simulink model "gantrycrane_animation2"  (Simulink 8.0)
settings: Solver=ode45  StartTime=0.0  StopTime=30  RelTol=1e-3
values from neighbouring files (symbols this model uses):
  kdth = -2*zetath*wnth*P.mc*P.L    [param.m]
  kdx = -0.0685    [param.m]
  kpth = (P.mc+P.m)*P.g - wnth^2*P.mc*P.L    [param.m]
  kpx = -0.0385    [param.m]
undefined symbols (not defined in the file or in its folder): drawGantryCrane
libraries: simulink x1
settings Model: Creator=nedward  LastModifiedBy=tmclain
settings DataIOCC: SignalLoggingSaveFormat=ModelDataLogs
settings DebuggingCC: FcnCallInpInsideContextMsg=UseLocalSettings
settings GRTTargetCC: CombineOutputUpdateFcns=off  GRTInterface=on

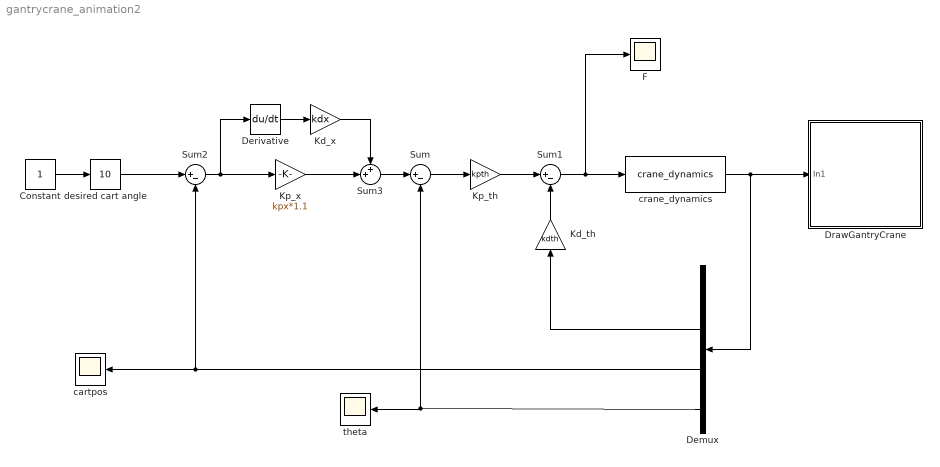
== system gantrycrane_animation2 ==
  Constant : Constant
  Demux : Demux
  Derivative : Derivative
  DrawGantryCrane : Subsystem
      mask init:
      | bar = 20;
      | crane = [5 3];
      | L1 = 10;
      | R1 = 1;
      mask Display: image(imread('tv.jpg'))
  F : Scope
      settings: TimeRange=30  YMin=-2000  YMax=14000  SaveName=ScopeData3
  Kd_th : Gain  Gain=kdth
  Kd_x : Gain  Gain=kdx
  Kp_th : Gain  Gain=kpth
  Kp_x : Gain  Gain=kpx*1.1
  Sum : Sum  Inputs=|+-
  Sum1 : Sum  Inputs=|+-
  Sum2 : Sum  Inputs=|+-
  Sum3 : Sum  Inputs=++|
  cartpos : Scope
      settings: TimeRange=30  YMin=0  YMax=12
  crane_dynamics : S-Function  FunctionName=crane_dynamics  Parameters=P  EnableBusSupport=off
  desired cart angle : simulink/Math Operations/Slider Gain  low=-10  gain=10  high=10
  theta : Scope
      settings: TimeRange=30  YMin=-0.2  YMax=0.15
  wires:
  crane_dynamics/1 -> DrawGantryCrane/1(In1), Demux/1
  Constant/1 -> desired cart angle/1
  Demux/2 -> Kd_th/1
  desired cart angle/1 -> Sum2/1
  Kd_th/1 -> Sum1/2
  Demux/4 -> theta/1, Sum/2
  Sum1/1 -> crane_dynamics/1, F/1
  Demux/3 -> cartpos/1, Sum2/2
  Kp_th/1 -> Sum1/1
  Sum/1 -> Kp_th/1
  Sum3/1 -> Sum/1
  Sum2/1 -> Kp_x/1, Derivative/1
  Kp_x/1 -> Sum3/2
  Derivative/1 -> Kd_x/1
  Kd_x/1 -> Sum3/1

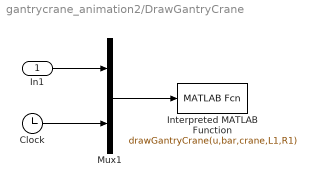
== system gantrycrane_animation2/DrawGantryCrane ==
  In1 : Inport
  Clock : Clock
  Interpreted MATLAB Function : MATLABFcn  MATLABFcn=drawGantryCrane(u,bar,crane,L1,R1)  OutputDimensions=0  SampleTime=0.1
  Mux1 : Mux  Inputs=2
  wires:
  Clock/1 -> Mux1/2
  Mux1/1 -> Interpreted MATLAB Function/1
  In1/1 -> Mux1/1
